simulink library "Propulsion_lib"  (R2020a)
settings: Solver=VariableStepAuto  StartTime=0.0  StopTime=10.0  RelTol=1e-3
undefined symbols (not defined in the file or in its folder): alphaf_deg, nr, nv, rho_reference_kgpm3, T_max, V_reference_mps, xf_m, zf_m
settings Model: Creator=muril  LastModifiedBy=muril

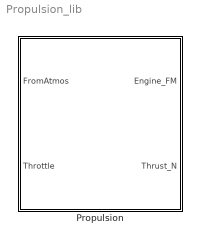
== system Propulsion_lib ==
  Propulsion : Subsystem

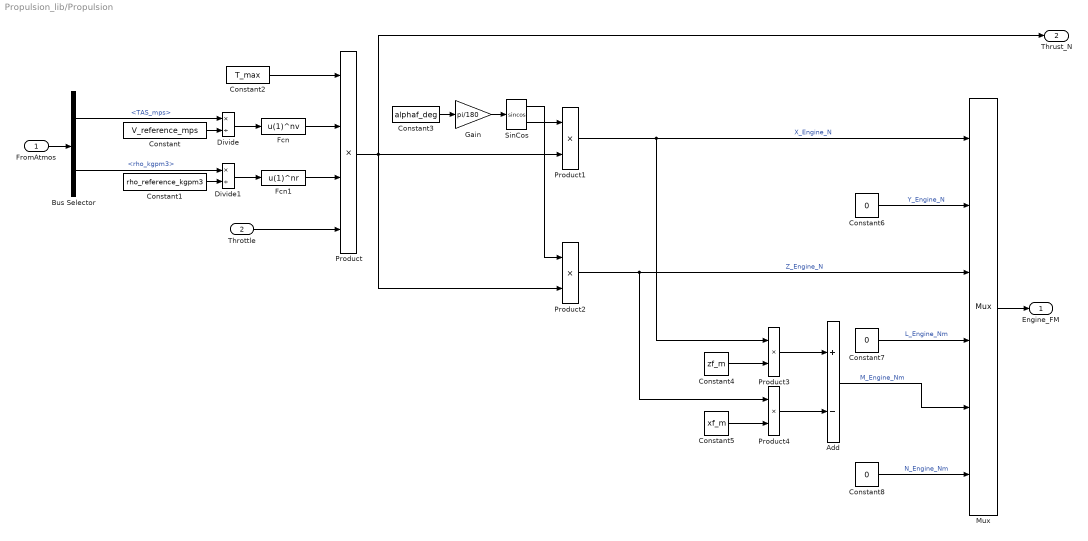
== system Propulsion_lib/Propulsion ==
  FromAtmos : Inport
  Throttle : Inport  Port=2
  Add : Sum  Inputs=+-
  Bus Selector : BusSelector  OutputSignals=TAS_mps,rho_kgpm3
  Constant : Constant  Value=V_reference_mps
  Constant1 : Constant  Value=rho_reference_kgpm3
  Constant2 : Constant  Value=T_max
  Constant3 : Constant  Value=alphaf_deg
  Constant4 : Constant  Value=zf_m
  Constant5 : Constant  Value=xf_m
  Constant6 : Constant  Value=0
  Constant7 : Constant  Value=0
  Constant8 : Constant  Value=0
  Divide : Product  Inputs=*/
  Divide1 : Product  Inputs=*/
  Fcn : Fcn  Expr=u(1)^nv
  Fcn1 : Fcn  Expr=u(1)^nr
  Gain : Gain  Gain=pi/180
  Mux : Mux  Inputs=6
  Product : Product  Inputs=4
  Product{1..4} (4 alike) : Product
  SinCos : Trigonometry  Operator=sincos
  Engine_FM : Outport
  Thrust_N : Outport  Port=2
  wires:
  SinCos/1 -> Product2/1
  Product4/1 -> Add/2
  Bus Selector/1 -> Divide/1  "<TAS_mps>"
  Product2/1 -> Product4/1, Mux/3  "Z_Engine_N"
  FromAtmos/1 -> Bus Selector/1
  Constant/1 -> Divide/2
  Mux/1 -> Engine_FM/1
  Product1/1 -> Product3/1, Mux/1  "X_Engine_N"
  Bus Selector/2 -> Divide1/1  "<rho_kgpm3>"
  Divide1/1 -> Fcn1/1
  Constant6/1 -> Mux/2  "Y_Engine_N"
  Product3/1 -> Add/1
  Divide/1 -> Fcn/1
  Product/1 -> Thrust_N/1, Product2/2, Product1/2
  Gain/1 -> SinCos/1
  Constant7/1 -> Mux/4  "L_Engine_Nm"
  Throttle/1 -> Product/4
  Constant1/1 -> Divide1/2
  Fcn/1 -> Product/2
  Fcn1/1 -> Product/3
  SinCos/2 -> Product1/1
  Constant8/1 -> Mux/6  "N_Engine_Nm"
  Constant2/1 -> Product/1
  Constant5/1 -> Product4/2
  Constant3/1 -> Gain/1
  Constant4/1 -> Product3/2
  Add/1 -> Mux/5  "M_Engine_Nm"
